simulink model "gotogoal"  (R2022b)
settings: Solver=VariableStepAuto  StartTime=0.0  StopTime=10.0  RelTol=1e-3
libraries: robotmobilelib x1
settings Model: Creator=hp  LastModifiedBy=hp

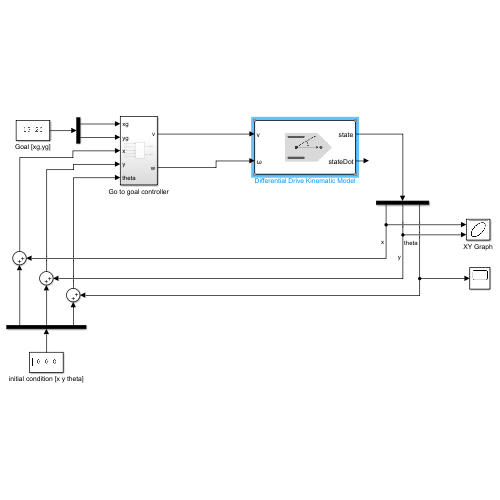
[thumbnail: Simulink's stored preview of the top-level diagram]
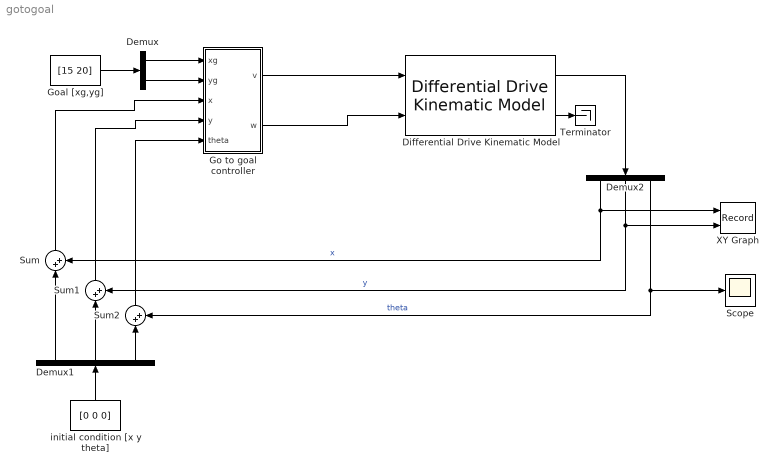
== system gotogoal ==
  Demux : Demux  Outputs=2
  Demux1 : Demux  Outputs=3
  Demux2 : Demux  Outputs=3
  Differential Drive Kinematic Model : robotmobilelib/Differential Drive Kinematic Model  VehicleInputs=Vehicle Speed & Heading Angular Velocity  WheelRadius=0.05  WheelSpeedRange=[-inf inf]  TrackWidth=0.35  InitialState=[0; 0; 0]  SimulateUsing=Interpreted execution
  Go to goal controller : Subsystem
  Goal [xg,yg] : Constant  Value=[15 20]
  Scope : Scope
  Sum : Sum  Inputs=|++
  Sum1 : Sum  Inputs=|++
  Sum2 : Sum  Inputs=|++
  Terminator : Terminator
  XY Graph : Record  FileSettingsInternal="{\"entries\":[{\"content\":{\"excelSettings\":{\"content\":{},\"type\":\"Streamout.ExcelSettings\"}},\"type\":\"Streamout.FileSettingStorage\",\"uuid\":\"b0bb26f3-d9e6-42e3-b8fd-46f1c4dfdefb\"}],\"packageUris\":[\"http://schema.mathworks.com/mf0/streamout_blocks/R2020a\"],\"version\":\"1.0\"}"  Layout=[1 1]  SignalsInternal="{\"entries\":[{\"content\":{\"signals\":[{\"content\":{\"blockPath\":[\"gotogoal/XY Graph\"],\"channel\":[],\"dimensions\":[1],\"domain\":\"gotogoal/XY Graph\",\"lineColor\":\"#a2142f\",\"plots\":[1],\"port\":1,\"sid\":[],\"signalID\":80,\"signalName\":\"x\"},\"type\":\"RecordBlkView.Signal\",\"uuid\":\"e2eeeb55-3116-49c4-a72d-551c5eeca17a\"},{\"content\":{\"blockPath\":[\"gotogoal/XY Graph\"],\"channel\":[],\"dimensions\":[1],\"domain\":\"gotogoal/XY Graph\",\"lineColor\":\"#139fff\",\"plots\":[1],\"port\":2,\"sid\":[],\"signalID\":83,\"signalName\":\"y\"},\"type\":\"RecordBlkView.Signal\",\"uuid\":\"e605a86f-9a8c-4267-a885-17e4451151ec\"}]},\"type\":\"RecordBlkView.InputSignals\",\"uuid\":\"80b72b32-e2aa-4d16-bb72-20eb3fcc2f01\"}],\"packageUris\":[\"http://schema.mathworks.com/mf0/streamout_blocks/R2020a\"],\"version\":\"1.0\"}"  VisualizationBindings="{\"xyplotplugin\":{\"info\":[{\"series\":[{\"bindingParametersList\":[{\"parameter\":\"X-Axis\",\"signalID\":80,\"signalName\":\"x\"},{\"parameter\":\"Y-Axis\",\"signalID\":83,\"signalName\":\"y\"}],\"seriesID\":17865}],\"subplotID\":1}]}}"  CompatibilityTag=XY
  initial condition [x y theta] : Constant  Value=[0 0 0]
  wires:
  Goal [xg,yg]/1 -> Demux/1
  Demux/1 -> Go to goal controller/1(xg)
  Demux/2 -> Go to goal controller/2(yg)
  Go to goal controller/1(v) -> Differential Drive Kinematic Model/1
  Go to goal controller/2(w) -> Differential Drive Kinematic Model/2
  initial condition [x y theta]/1 -> Demux1/1
  Demux1/1 -> Sum/1
  Demux1/2 -> Sum1/1
  Demux1/3 -> Sum2/1
  Differential Drive Kinematic Model/1 -> Demux2/1
  Demux2/1 -> XY Graph/1, Sum/2  "x"
  Demux2/2 -> XY Graph/2, Sum1/2  "y"
  Demux2/3 -> Sum2/2, Scope/1  "theta"
  Sum/1 -> Go to goal controller/3(x)
  Sum1/1 -> Go to goal controller/4(y)
  Sum2/1 -> Go to goal controller/5(theta)
  Differential Drive Kinematic Model/2 -> Terminator/1

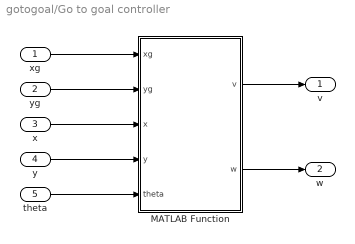
== system gotogoal/Go to goal controller ==
  xg : Inport
  yg : Inport  Port=2
  x : Inport  Port=3
  y : Inport  Port=4
  theta : Inport  Port=5
  MATLAB Function : MATLAB Function  TreatAsAtomicUnit=on
  v : Outport
  w : Outport  Port=2
  wires:
  xg/1 -> MATLAB Function/1(xg)
  yg/1 -> MATLAB Function/2(yg)
  x/1 -> MATLAB Function/3(x)
  y/1 -> MATLAB Function/4(y)
  theta/1 -> MATLAB Function/5(theta)
  MATLAB Function/1(v) -> v/1
  MATLAB Function/2(w) -> w/1

== matlab function gotogoal/Go to goal controller/MATLAB Function ==
  data: xg input; v output; w output; yg input; x input; y input; theta input
function [v, w] = fcn(xg, yg, x, y, theta)
    % Go-to-Goal Kontrolcüsü
    % Girişler:
    %   xg, yg - Hedef (goal) konum
    %   x, y   - Robotun mevcut (initial) konumu
    %   theta  - Robotun mevcut yönelimi (radyan cinsinden)
    % Çıkışlar:
    %   v      - Doğrusal hız
    %   w      - Açısal hız

    
    Kp = 0.5;   % Hedefe olan mesafe için kazanç
    Kh = 1.5;   % Hedefe olan açısal hata için kazanç

    mesafe = sqrt((xg - x)^2 + (yg - y)^2);
    alpha = atan2(yg - y, xg - x) - theta;

    v = Kp * mesafe;
    w = Kh * alpha;

    if mesafe < 0.1
        v = 0;
        w = 0;
    end
end
